simulink model "rtwdemo_basicsc"  (Simulink 6.0)
settings: Solver=FixedStepDiscrete  StartTime=0.0  StopTime=10.0  RelTol=1e-3
PostLoadFcn:
  | open_system('rtwdemo_basicsc/Auto');
values from neighbouring files (symbols this model uses):
  LOWER = Simulink.Parameter    [rtwdemo_exprfolding_data.m]
  T1Break = Simulink.Parameter    [rtwdemo_exprfolding_data.m]    (also in rtwdemo_paraminline_data.m; rtwdemo_ssreuse_data.m)
  T1Data = Simulink.Parameter    [rtwdemo_exprfolding_data.m]    (also in rtwdemo_paraminline_data.m; rtwdemo_ssreuse_data.m)
  T2Data = Simulink.Parameter    [rtwdemo_exprfolding_data.m]    (also in rtwdemo_paraminline_data.m; rtwdemo_ssreuse_data.m = copy(T1Data))
  UPPER = Simulink.Parameter    [rtwdemo_exprfolding_data.m]
undefined symbols (not defined in the file or in its folder): K1
libraries: rtwdemowidgets x2
settings Model: CovMetricSettings=d  Creator=The MathWorks Inc.  LastModifiedBy=batserve  ExtModeAutoUpdateStatusClock=off
settings DataIOCC: SignalLoggingName=sigsOut
settings OptimizationCC: InlineParams=on  EnforceIntegerDowncast=off  StateBitsets=on  DataBitsets=on  UseTempVars=on
settings DebuggingCC: CheckExecutionContextPreStartOutputMsg=on  CheckExecutionContextRuntimeOutputMsg=on  SignalResolutionControl=UseLocalSettings  SolverPrmCheckMsg=none
settings RTWCC: TLCOptions=-p0  GenerateReport=on  RTWVerbose=off  ProcessScript=grt_make_rtw_hook  LaunchReport=on
settings CodeAppCC: PrefixModelToSubsysFcnNames=off

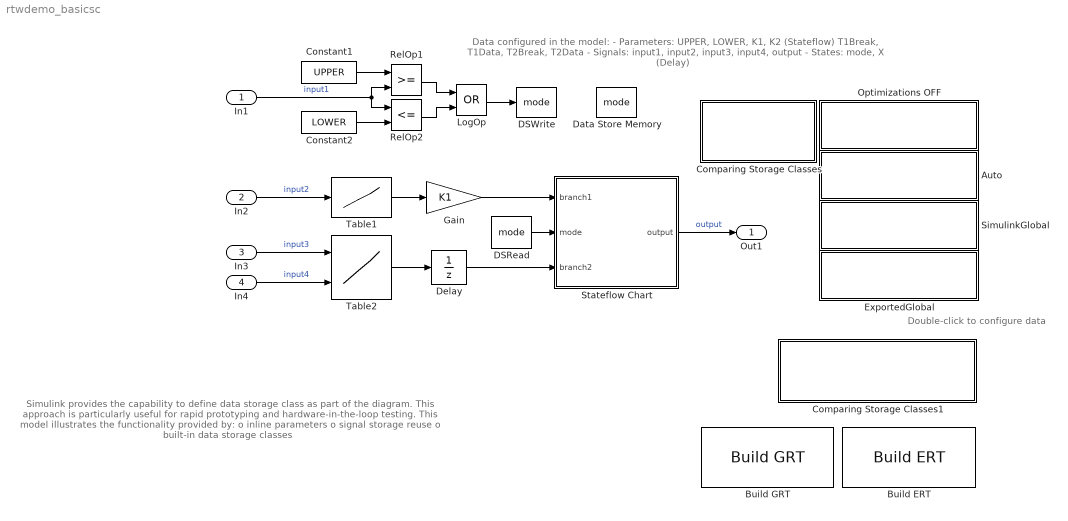
== system rtwdemo_basicsc ==
  note: Data configured in the model:
      | - Parameters: UPPER, LOWER, K1, K2 (Stateflow)
      |   T1Break, T1Data, T2Break, T2Data
      | - Signals: input1, input2, input3, input4, output
      | - States: mode, X (Delay)
  note: Double-click to configure data
  note: Simulink provides the capability to define data storage class as part of
      | the diagram. This approach is particularly useful for rapid prototyping
      | and hardware-in-the-loop testing.
      |
      | This model illustrates the functionality provided by:
      | o inline parameters
      | o signal storage reuse
      | o built-in data storage classes
  In1 : Inport  Port=1  PortDimensions=1  SampleTime=1  LatchInput=off
  In2 : Inport  Port=2  PortDimensions=1  LatchInput=off
  In3 : Inport  Port=3  PortDimensions=1  LatchInput=off
  In4 : Inport  Port=4  PortDimensions=1  LatchInput=off
  Auto : Subsystem  PropExecContextAcrossSSBoundary=on  mask(Basic data packaging - configure model){Optimizations=on, StorageClass=Auto, DataInitFcn=rtwdemo_basicsc_config}
      mask prompts: Optimizations "Use Optimizations"
      mask help: OpenFcn configures model for data packaging demo.
      mask init:
      | if strcmp(Optimizations, 'on')
      |   dispStr = [StorageClass, '\nStorage Class'];
      | else
      |   set_param(gcb, 'StorageClass', 'Auto');
      |   dispStr = ['InlineParameters OFF\n', ...
      | 		     'SignalStorageReuse OFF'];
      | end
      settings: OpenFcn=feval(get_param(gcb, 'DataInitFcn'), bdroot(gcb), get_param(gcb, 'Optimizations'), get_param(gcb, 'StorageClass'));
      mask StyleString: checkbox,popup(Auto|SimulinkGlobal|ExportedGlobal),edit
      mask CallbackString:
      | if strcmp(get_param(gcb, 'Optimizations'), 'off')
      |   set_param(gcb, 'MaskEnableString', 'on,off,on');
      | else
      |   set_param(gcb, 'MaskEnableString', 'on,on,on');
      | end||
      mask Display: disp(dispStr);
  Build ERT : rtwdemowidgets/Build ERT  attrib_overrides={}
  Build GRT : rtwdemowidgets/Build GRT  attrib_overrides={}
  Comparing Storage Classes : Subsystem  PropExecContextAcrossSSBoundary=on
      mask Display: disp(['Compare the\noptions ..', '.\n(double-click)']);
  Comparing Storage Classes1 : Subsystem  PropExecContextAcrossSSBoundary=on
      settings: OpenFcn=rtwdemo_advsc
      mask Display: disp(['Advanced data packaging using\nSimulink data objects ..', '.\n(double-click)']);
  Constant1 : Constant  Value=UPPER
  Constant2 : Constant  Value=LOWER
  DSRead : DataStoreRead  DialogController=Simulink.DDGSource  DataStoreName=mode  SampleTime=1
  DSWrite : DataStoreWrite  DialogController=Simulink.DDGSource  DataStoreName=mode  SampleTime=-1
  Data Store Memory : DataStoreMemory  DialogController=Simulink.DDGSource  DataStoreName=mode  InitialValue=0
  Delay : UnitDelay  StateIdentifier=X
  ExportedGlobal : Subsystem  PropExecContextAcrossSSBoundary=on  mask(Basic data packaging - configure model){Optimizations=on, StorageClass=ExportedGlobal, DataInitFcn=rtwdemo_basicsc_config}
      mask prompts: Optimizations "Use Optimizations"
      mask help: OpenFcn configures model for data packaging demo.
      mask init: same as rtwdemo_basicsc/Auto
      settings: OpenFcn=feval(get_param(gcb, 'DataInitFcn'), bdroot(gcb), get_param(gcb, 'Optimizations'), get_param(gcb, 'StorageClass'));
      mask StyleString: checkbox,popup(Auto|SimulinkGlobal|ExportedGlobal),edit
      mask CallbackString:
      | if strcmp(get_param(gcb, 'Optimizations'), 'off')
      |   set_param(gcb, 'MaskEnableString', 'on,off,on');
      | else
      |   set_param(gcb, 'MaskEnableString', 'on,on,on');
      | end||
      mask Display: disp(dispStr);
  Gain : Gain  Gain=K1  SaturateOnIntegerOverflow=on
  LogOp : Logic  Operator=OR
  Optimizations OFF : Subsystem  PropExecContextAcrossSSBoundary=on  mask(Basic data packaging - configure model){Optimizations=off, StorageClass=Auto, DataInitFcn=rtwdemo_basicsc_config}
      mask prompts: Optimizations "Use Optimizations"
      mask help: OpenFcn configures model for data packaging demo.
      mask init: same as rtwdemo_basicsc/Auto
      settings: OpenFcn=feval(get_param(gcb, 'DataInitFcn'), bdroot(gcb), get_param(gcb, 'Optimizations'), get_param(gcb, 'StorageClass'));
      mask StyleString: checkbox,popup(Auto|SimulinkGlobal|ExportedGlobal),edit
      mask CallbackString:
      | if strcmp(get_param(gcb, 'Optimizations'), 'off')
      |   set_param(gcb, 'MaskEnableString', 'on,off,on');
      | else
      |   set_param(gcb, 'MaskEnableString', 'on,on,on');
      | end||
      mask Display: disp(dispStr);
  RelOp1 : RelationalOperator  InputSameDT=on
  RelOp2 : RelationalOperator  Operator=<=  InputSameDT=on
  SimulinkGlobal : Subsystem  PropExecContextAcrossSSBoundary=on  mask(Basic data packaging - configure model){Optimizations=on, StorageClass=SimulinkGlobal, DataInitFcn=rtwdemo_basicsc_config}
      mask prompts: Optimizations "Use Optimizations"
      mask help: OpenFcn configures model for data packaging demo.
      mask init: same as rtwdemo_basicsc/Auto
      settings: OpenFcn=feval(get_param(gcb, 'DataInitFcn'), bdroot(gcb), get_param(gcb, 'Optimizations'), get_param(gcb, 'StorageClass'));
      mask StyleString: checkbox,popup(Auto|SimulinkGlobal|ExportedGlobal),edit
      mask CallbackString:
      | if strcmp(get_param(gcb, 'Optimizations'), 'off')
      |   set_param(gcb, 'MaskEnableString', 'on,off,on');
      | else
      |   set_param(gcb, 'MaskEnableString', 'on,on,on');
      | end||
      mask Display: disp(dispStr);
  Stateflow Chart : Stateflow chart  PropExecContextAcrossSSBoundary=on
      settings: PermitHierarchicalResolution=ParametersOnly
  Table1 : Lookup  DialogController=Simulink.DDGSource  InputValues=T1Break  OutputValues=T1Data  SaturateOnIntegerOverflow=on
  Table2 : Lookup2D  DialogController=Simulink.DDGSource  RowIndex=T2Break  ColumnIndex=T2Break  OutputValues=T2Data  OutScaling=2^-10  InputSameDT=on
  Out1 : Outport
  wires:
  RelOp1/1 -> LogOp/1
  RelOp2/1 -> LogOp/2
  Constant2/1 -> RelOp2/2
  In2/1 -> Table1/1  "input2"
  Gain/1 -> Stateflow Chart/1(branch1)
  Table1/1 -> Gain/1
  Table2/1 -> Delay/1
  Constant1/1 -> RelOp1/1
  In1/1 -> RelOp1/2, RelOp2/1  "input1"
  In3/1 -> Table2/1  "input3"
  In4/1 -> Table2/2  "input4"
  Stateflow Chart/1(output) -> Out1/1  "output"
  Delay/1 -> Stateflow Chart/3(branch2)
  LogOp/1 -> DSWrite/1
  DSRead/1 -> Stateflow Chart/2(mode)

== system rtwdemo_basicsc/Auto ==

== system rtwdemo_basicsc/Comparing Storage Classes ==
  note: 4. Unstructured storage classes (e.g., ExportedGlobal):
      |
      | Motivation:
      | - Interface to global data in hand-written (legacy) code
      |
      | Behavior:
      | - Select parameters and signals are global, unstructured variables
      | - Select states and root-level I/O are global, unstructured variables
      |
      | Advantages:
      | - Data names are preserved in the generated code
      |
      | Disadvantages:
      | - Imposes certain modeling restrictions
      | - Disables certain code optimizations
  note: 3. SimulinkGlobal storage class:
      |
      | Motivation:
      | - Provide visibility (persistence) for selected data
      |
      | Behavior:
      | - Select parameters and signals are members of persistent data structures
      | - All states and root-level I/O are members of persistent data structures
      |
      | Advantages:
      | - Only increase memory usage for data of interest
      | - Provides visibility to data without limitations
      |
      | Disadvantages:
      | - Minimal control over variable names
      |
      | How to specify SimulinkGlobal:
      | - Parameters: Tunable + Auto storage class
      | - Signals: Test point + Auto storage class
      | - States: Auto storage class
  note: 2. Auto storage class:
      |
      | Motivation:
      | - Maximize efficiency of the generated code
      |
      | Behavior:
      | - Parameters are inlined and intermediate signals are eliminated
      | - All states and root-level I/O are members of persistent data structures
      |
      | Advantages:
      | - Optimized code generation
      | - Default behavior when optimizations enabled (easy to use)
      |
      | Disadvantages:
      | - Parameters and signals do not appear as variables in the generated code
  note: 1. Inline parameters and signal storage reuse OFF:
      |
      | Motivation:
      | - Provide visibility (persistence) for all data
      | - Useful for simulation and rapid prototyping
      |
      | Behavior:
      | - All parameters and signals are members of persistent data structures
      | - All states and root-level I/O are members of persistent data structures
      |
      | Advantages:
      | - Easy access to data via model-wide settings
      |
      | Disadvantages:
      | - Generated code is non-optimal
      | - Minimal control over variable names
  note: NOTE: Descriptions 2-4 assume that the inline parameters and signal storage reuse optimizations are ON.

== system rtwdemo_basicsc/Comparing Storage Classes1 ==

== system rtwdemo_basicsc/ExportedGlobal ==

== system rtwdemo_basicsc/Optimizations OFF ==

== system rtwdemo_basicsc/SimulinkGlobal ==

== stateflow chart Stateflow Chart ==
  note: This chart is acting as an if-else condition,
      |     with the result multiplied by K2.
      | Using a Simulink switch (or if-action) and gain block,
      |     results in virtually identical code.
  (junction 7) -> (junction 4) : {output = branch1;}
  (junction 4) -> (junction 6) : {output *= K2;}
  (junction 5) -> (junction 4) : {output = branch2;}
  (default) -> (junction 5)
  (junction 5) -> (junction 7) : [mode]
  data: branch1 input double size=1; mode input boolean size=1; branch2 input double size=1; output output double size=1; K2 parameter double size=1
